simulink model "Lab5_2017B5A30983P"  (R2019b)
settings: Solver=ode45  StartTime=0.0  StopTime=0.1  RelTol=1e-3
libraries: powerlib x10
settings Model: Creator=swaga  LastModifiedBy=swaga

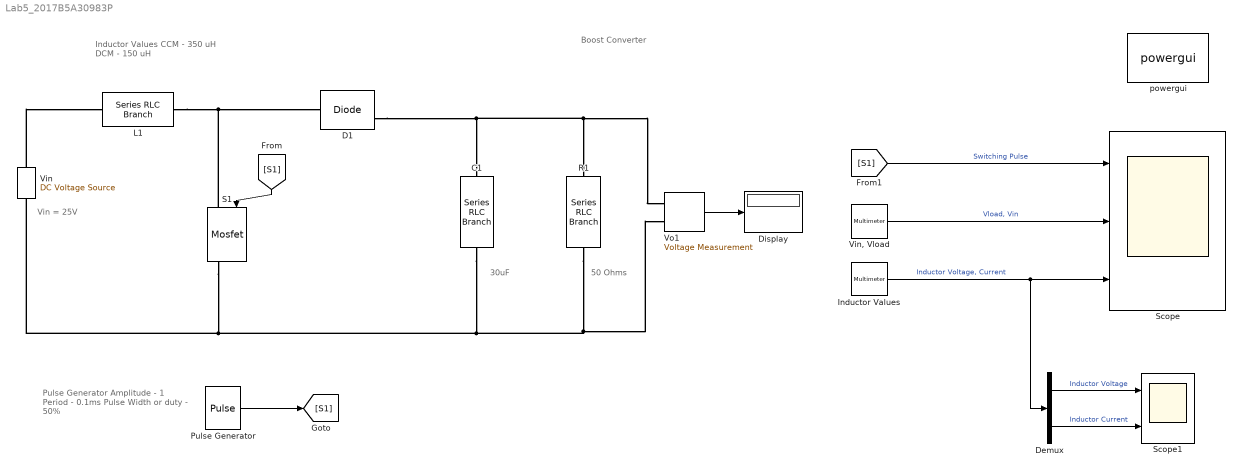
== system Lab5_2017B5A30983P ==
  note: Boost Converter
  note: Pulse Generator
      | Amplitude - 1
      | Period - 0.1ms
      | Pulse Width or duty - 50%
  note: Inductor Values
      | CCM - 350 uH
      | DCM - 150 uH
  note: Vin = 25V
  note: 50 Ohms
  note: 30uF
  C1 : powerlib/Elements/Series RLC Branch  LConnTagsString=__new0  RConnTagsString=__new0  BranchType=C  Resistance=1  Inductance=1e-3  SetiL0=off  InitialCurrent=0  Capacitance=30e-6  Setx0=off  InitialVoltage=0  Measurements=None
      settings: SourceProductName=Simscape Electrical
  D1 : powerlib/Power Electronics/Diode  Ron=0.001  Lon=0  Vf=0.8  IC=0  UseSnubber=0  Rs=500  Cs=250e-9  Measurements=on
      settings: SourceProductName=Simscape Electrical
  Demux : Demux  Outputs=2
  Display : Display
  "Inductor Values " : powerlib/Measurements/Multimeter  PhasorSimulation=off  OutputType=Complex  sel=[1 4]  L=4  Gain=[1 1]  yselected={'Ub: L1','Ib: L1'};  PSBOutputType=1  PSBequivalent=0  AxesSetting=[0,0.1,-100,100]  Display=0  SavedBlockNames=-11
      settings: SourceProductName=Simscape Electrical
  L1 : powerlib/Elements/Series RLC Branch  LConnTagsString=__new0  RConnTagsString=__new0  BranchType=L  Resistance=1  Inductance=150e-6  SetiL0=off  InitialCurrent=0  Capacitance=1e-6  Setx0=off  InitialVoltage=0  Measurements=Branch voltage and current
      settings: SourceProductName=Simscape Electrical
  "Pulse Generator " : DiscretePulseGenerator  PulseType=Time based  Period=1e-4  PulseWidth=50
  R1 : powerlib/Elements/Series RLC Branch  LConnTagsString=__new0  RConnTagsString=__new0  BranchType=R  Resistance=50  Inductance=1e-3  SetiL0=off  InitialCurrent=0  Capacitance=1e-6  Setx0=off  InitialVoltage=0  Measurements=Branch voltage
      settings: SourceProductName=Simscape Electrical
  S1 : powerlib/Power Electronics/Mosfet  Ron=0.1  Lon=0  Rd=0.01  Vfd=0  IC=0  Rs=3.5e-9  Cs=3.5e-9  Measurements=on
      settings: SourceProductName=Simscape Electrical
  Scope : Scope  NumInputPorts=3
  Scope1 : Scope  NumInputPorts=2
  Vin : powerlib/Electrical Sources/DC Voltage Source  Amplitude=25  Measurements=Voltage
      settings: SourceProductName=Simscape Electrical
  "Vin, Vload" : powerlib/Measurements/Multimeter  PhasorSimulation=off  OutputType=Complex  sel=[2 3]  L=4  Gain=[1 1]  yselected={'Ub: R1','Usrc: Vin'};  PSBOutputType=1  PSBequivalent=0  AxesSetting=[0,0.1,-100,100]  Display=0  SavedBlockNames=-11
      settings: SourceProductName=Simscape Electrical
  Vo1 : powerlib/Measurements/Voltage Measurement  PhasorSimulation=off  OutputType=Complex  PSBequivalent=0
      settings: SourceProductName=Simscape Electrical
  "powergui " : powerlib/powergui  Priority=1  SimulationMode=Discrete  SampleTime=2.5e-7  frequency=60  Iterations=50  frequencyindice=0  Pbase=100e6  ErrMax=1e-4  UnitsV=kV  UnitsW=MW  buscounter=0  FunctionMessages=off  echomessages=off  EnableUseOfTLC=off  CurrentSourceSwitches=off  DisableSnubberDevices=off  DisableRonSwitches=off  DisableVfSwitches=off  DisplayEquations=off  AutomaticDiscreteSolvers=off  SolverType=Tustin/Backward Euler (TBE)  Interpol=off  ExternalGateDelay=off  methode=off  Ts=100  x0status=blocks  SPID=on  SwTol=0  HookPort=off  NonlinearTolerance=1e-4  nMaxIteration=100  ContinueOnMaxIteration=off  RestoreLinks=warning  ResistiveCurrentMeasurement=off  Frange=[0:2:500]  Ylog=off  Xlog=on  ShowGrid=off  save=off  variable=ZData  structure=0  ZoomFFT=off  StartTime=0.0  cycles=1  DisplayStyle=1  fundamental=60  FreqAxis=off  MaxFrequency=1000  frequencyindicesteady=1  RmsSteady=1  display=off
      settings: SourceProductName=Simscape Electrical
  wires:
  [S1] -> Scope/1  "Switching Pulse"
  Vo1/1 -> Display/1
  "Pulse Generator "/1 -> [S1]
  "Inductor Values "/1 -> Demux/1, Scope/3  "Inductor Voltage, Current"
  "Vin, Vload"/1 -> Scope/2  "Vload, Vin"
  [S1] -> S1/1
  Demux/1 -> Scope1/1  "Inductor Voltage"
  Demux/2 -> Scope1/2  "Inductor Current"
  connections:
  C1/RConn1 -- Vo1/LConn2 -- R1/RConn1 -- S1/RConn1 -- Vin/LConn1
  Vo1/LConn1 -- R1/LConn1 -- D1/RConn1 -- C1/LConn1
  Vin/RConn1 -- L1/LConn1
  L1/RConn1 -- S1/LConn1 -- D1/LConn1
